simulink model "PubIfDecisionVSM_UOM"  (R2020b)
settings: Solver=FixedStepAuto  StartTime=0.0  StopTime=Inf  RelTol=1e-3
PostLoadFcn:
  | if any(exist('dsrtsu_mdlpostloadfcn', 'file') ~= 0), dsrtsu_mdlpostloadfcn('Execute', bdroot); end
InitFcn:
  | , if any(exist('dsmpb_private', 'file') ~= 0), dsmpb_private('dsmpb_mdlclblib', 'Init', bdroot); end,
PreSaveFcn:
  | , if any(exist('dsmpb_private', 'file') ~= 0), dsmpb_private('dsmpb_mdlclblib', 'PreSave', bdroot); end,
CloseFcn:
  | , if any(exist('dsmpb_private', 'file') ~= 0), dsmpb_private('dsmpb_mdlclblib', 'Close', bdroot); end,
settings Model: DataDictionary=HWA_DDs.sldd  RTICANMMDATA=struct('GeneralSetupData',struct('modelroot','E:\V71\Model\ADAS_Store\Adas\VSM\UOM','generalsettings',struct('filesettings',struct('destfolder',struct('Name','RTICANMM_FILES','Check',1),'buildfolder',struct('Name','.','Check',1),'AbsDestfolder',struct('Name','E:\V71\Model\ADAS_Store\Adas\VSM\UOM\RTICANMM_FILES'),'AbsBuildfolder',struct('Name','E:\V71\Model\ADAS_Store\Adas\VSM\UOM'))),'options',struct('addpaths',1,'rmpaths',1,'addtrcexclusion',false,'cannavigator',struct('checkmonitoring',0),'show_usrtrc',0,'use_usrtrc',0),'advanced',struct('options',ones(1,100)),'MPSetup',{{}},'RTI',struct('Type','DSRT','Ver','4.2','Date','02-Nov-2019'),'modelname','PubIfDecisionVSM_UOM','block','PubIfDecisionVSM_UOM'))  DSRTSU_INTERNAL_RTIFPGA=150  Creator=GW00180895  LastModifiedBy=GW00208968
settings OptimizationCC: BlockReduction=off  ConditionallyExecuteInputs=off  OptimizeBlockIOStorage=off  BufferReuse=off  GlobalBufferReuse=off  ExpressionFolding=off  LocalBlockOutputs=off  OptimizeDataStoreBuffers=off  BusAssignmentInplaceUpdate=off
settings DebuggingCC: TasksWithSamePriorityMsg=none
settings HardwareCC: ProdBitPerPointer=32  ProdBitPerSizeT=32  ProdBitPerPtrDiffT=32  ProdLargestAtomicInteger=Integer  ProdWordSize=32  ProdHWDeviceType=Custom Processor->Custom
settings ModelReferenceCC: UpdateModelReferenceTargets=IfOutOfDate  EnableParallelModelReferenceBuilds=on  ModelReferenceNumInstancesAllowed=Single
settings SFSimCC: MATLABDynamicMemAlloc=off
settings RTWCC: Description=dSPACE Run-Time Target (for VEOS on Windows and ConfigurationDesk)  SystemTargetFile=dsrt.tlc  GenCodeOnly=on  MakeCommand=make_dsrt  TemplateMakefile=dsrt_default_tmf  RTWVerbose=off
settings STFCustomTargetCC: TargetLangStandard=C99 (ISO)  ParMdlRefBuildCompliant=on  ConcurrentExecutionCompliant=off  CPPClassGenCompliant=off  GRTInterface=off  SystemTargetFile=dsrt.tlc
settings GRTTargetCC: CompOptLevelCompliant=off  ConcurrentExecutionCompliant=off  CombineOutputUpdateFcns=off  MatFileLogging=off  CPPClassGenCompliant=off  UseToolchainInfoCompliant=off

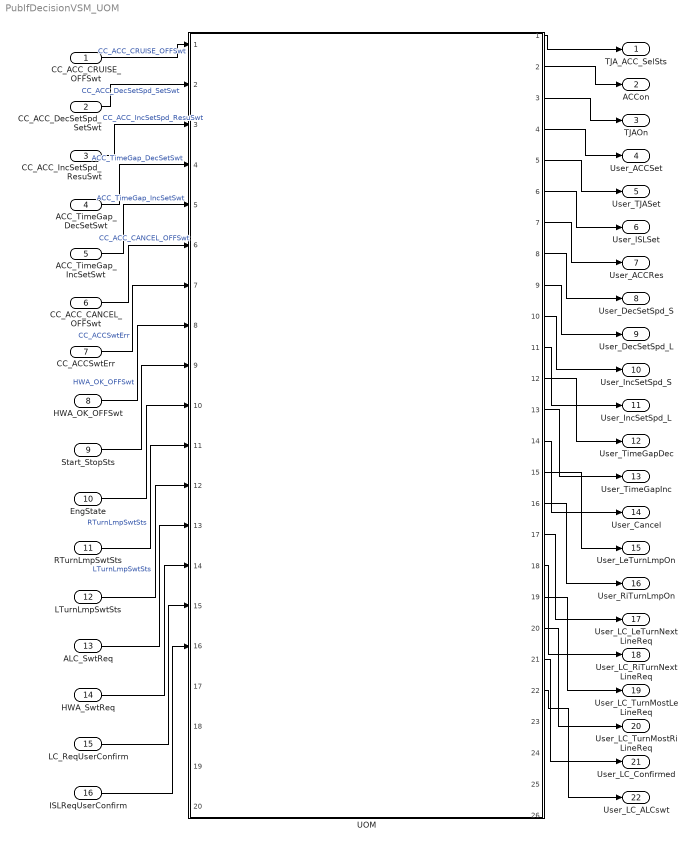
== system PubIfDecisionVSM_UOM ==
  CC_ACC_CRUISE_OFFSwt : Inport  OutDataTypeStr=boolean  PortDimensions=1
  CC_ACC_DecSetSpd_SetSwt : Inport  Port=2  OutDataTypeStr=boolean  PortDimensions=1
  CC_ACC_IncSetSpd_ResuSwt : Inport  Port=3  OutDataTypeStr=boolean  PortDimensions=1
  ACC_TimeGap_DecSetSwt : Inport  Port=4  OutDataTypeStr=boolean  PortDimensions=1
  ACC_TimeGap_IncSetSwt : Inport  Port=5  OutDataTypeStr=boolean  PortDimensions=1
  CC_ACC_CANCEL_OFFSwt : Inport  Port=6  OutDataTypeStr=boolean  PortDimensions=1
  CC_ACCSwtErr : Inport  Port=7  OutDataTypeStr=boolean  PortDimensions=1
  HWA_OK_OFFSwt : Inport  Port=8  OutDataTypeStr=boolean  PortDimensions=1
  Start_StopSts : Inport  Port=9  OutDataTypeStr=uint8
  EngState : Inport  Port=10  OutDataTypeStr=uint8
  RTurnLmpSwtSts : Inport  Port=11  OutDataTypeStr=boolean  PortDimensions=1
  LTurnLmpSwtSts : Inport  Port=12  OutDataTypeStr=boolean  PortDimensions=1
  ALC_SwtReq : Inport  Port=13  OutDataTypeStr=boolean
  HWA_SwtReq : Inport  Port=14  OutDataTypeStr=boolean
  LC_ReqUserConfirm : Inport  Port=15  OutDataTypeStr=boolean
  ISLReqUserConfirm : Inport  Port=16  OutDataTypeStr=boolean
  UOM : Subsystem  ReferencedSubsystem=PvtSubSys_VSM_UOM
  TJA_ACC_SelSts : Outport  OutDataTypeStr=uint8
  ACCon : Outport  Port=2  OutDataTypeStr=boolean
  TJAOn : Outport  Port=3  OutDataTypeStr=boolean
  User_ACCSet : Outport  Port=4  OutDataTypeStr=boolean
  User_TJASet : Outport  Port=5  OutDataTypeStr=boolean
  User_ISLSet : Outport  Port=6  OutDataTypeStr=boolean
  User_ACCRes : Outport  Port=7  OutDataTypeStr=boolean
  User_DecSetSpd_S : Outport  Port=8  OutDataTypeStr=boolean
  User_DecSetSpd_L : Outport  Port=9  OutDataTypeStr=boolean
  User_IncSetSpd_S : Outport  Port=10  OutDataTypeStr=boolean
  User_IncSetSpd_L : Outport  Port=11  OutDataTypeStr=boolean
  User_TimeGapDec : Outport  Port=12  OutDataTypeStr=boolean
  User_TimeGapInc : Outport  Port=13  OutDataTypeStr=boolean
  User_Cancel : Outport  Port=14  OutDataTypeStr=boolean
  User_LeTurnLmpOn : Outport  Port=15  OutDataTypeStr=boolean
  User_RiTurnLmpOn : Outport  Port=16  OutDataTypeStr=boolean
  User_LC_LeTurnNextLineReq : Outport  Port=17  OutDataTypeStr=boolean
  User_LC_RiTurnNextLineReq : Outport  Port=18  OutDataTypeStr=boolean
  User_LC_TurnMostLeLineReq : Outport  Port=19  OutDataTypeStr=boolean
  User_LC_TurnMostRiLineReq : Outport  Port=20  OutDataTypeStr=boolean
  User_LC_Confirmed : Outport  Port=21  OutDataTypeStr=boolean
  User_LC_ALCswt : Outport  Port=22  OutDataTypeStr=uint8
  wires:
  UOM/22 -> User_LC_ALCswt/1
  UOM/17 -> User_LC_LeTurnNextLineReq/1
  UOM/19 -> User_LC_TurnMostLeLineReq/1
  UOM/20 -> User_LC_TurnMostRiLineReq/1
  UOM/21 -> User_LC_Confirmed/1
  UOM/18 -> User_LC_RiTurnNextLineReq/1
  UOM/2 -> ACCon/1
  UOM/7 -> User_ACCRes/1
  LC_ReqUserConfirm/1 -> UOM/15
  UOM/12 -> User_TimeGapDec/1
  UOM/16 -> User_RiTurnLmpOn/1
  UOM/15 -> User_LeTurnLmpOn/1
  UOM/14 -> User_Cancel/1
  UOM/1 -> TJA_ACC_SelSts/1
  UOM/13 -> User_TimeGapInc/1
  UOM/11 -> User_IncSetSpd_L/1
  UOM/4 -> User_ACCSet/1
  UOM/10 -> User_IncSetSpd_S/1
  UOM/9 -> User_DecSetSpd_L/1
  ACC_TimeGap_IncSetSwt/1 -> UOM/5  "ACC_TimeGap_IncSetSwt"
  HWA_OK_OFFSwt/1 -> UOM/8  "HWA_OK_OFFSwt"
  UOM/6 -> User_ISLSet/1
  UOM/5 -> User_TJASet/1
  UOM/8 -> User_DecSetSpd_S/1
  UOM/3 -> TJAOn/1
  HWA_SwtReq/1 -> UOM/14
  ISLReqUserConfirm/1 -> UOM/16
  ALC_SwtReq/1 -> UOM/13
  LTurnLmpSwtSts/1 -> UOM/12  "LTurnLmpSwtSts"
  RTurnLmpSwtSts/1 -> UOM/11  "RTurnLmpSwtSts"
  CC_ACCSwtErr/1 -> UOM/7  "CC_ACCSwtErr"
  Start_StopSts/1 -> UOM/9
  ACC_TimeGap_DecSetSwt/1 -> UOM/4  "ACC_TimeGap_DecSetSwt"
  EngState/1 -> UOM/10
  CC_ACC_CANCEL_OFFSwt/1 -> UOM/6  "CC_ACC_CANCEL_OFFSwt"
  CC_ACC_IncSetSpd_ResuSwt/1 -> UOM/3  "CC_ACC_IncSetSpd_ResuSwt"
  CC_ACC_DecSetSpd_SetSwt/1 -> UOM/2  "CC_ACC_DecSetSpd_SetSwt"
  CC_ACC_CRUISE_OFFSwt/1 -> UOM/1  "CC_ACC_CRUISE_OFFSwt"
